simulink model "save_old_atan2"  (Simulink 7.6)
settings: Solver=ode45  StartTime=0.0  StopTime=10.0  RelTol=1e-3
libraries: simulink x14
settings Model: Creator=jporter  LastModifiedBy=jporter

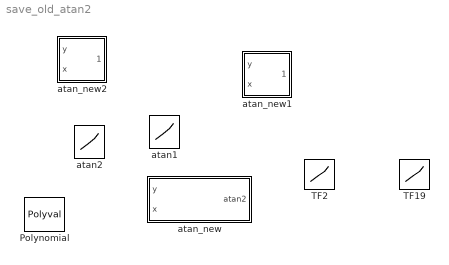
== system save_old_atan2 ==
  Polynomial : Polyval  Coefs=polyfit( [-100:100], atan( [-100:100] ), 12 )
  TF19 : Lookup  InputValues=[-5:5]  Table=atan([-5:5])  OutDataTypeStr=double
  TF2 : Lookup  InputValues=fi([-10 -5 -2.5:.1:-.11 -.1:.001:.1 .11:.1:2.5 5 10], 1, 32, 27)  Table=fi([ -pi/2 atan([-5 -2.5:.1:-.11 -.1:.001:.1 .11:.1:2.5 5]) pi/2 ], 1, 32, 30)  LookUpMeth=Interpolation-Use End Values  OutDataTypeStr=double
  atan1 : Lookup2D  RowIndex=[-0.0007 -7e-005 -7e-006 -7e-007 -7e-008 0 7e-008 7e-007 7e-006 7e-005 0.0007]  ColumnIndex=[-0.0004 -4e-005 -4e-006 -4e-007 -4e-008 0 4e-008 4e-007 4e-006 4e-005 0.0004]  Table=[-2.08994244104142 -1.62787710920116 -1.57651055031409 -1.57136775530413 -1.57085346965198 -1.5707963267949 -1.57073918393782 -1.57022489828566 -1.5650821032757 -1.51371554438863 -1.05165021254837;-2.96834698713743 -2.08994244104142 -1.62787710920116 -1.57651055031409 -1.57136775530413 -1.5707963267949 -1.57022489828566 -1.5650821032757 -1.51371554438863 -1.05165021254837 -0.173245666452365;-3.12409443971994 -2.96834698713743 -2.08994244104142 -1.62787710920116 -1.57651055031409 -1.5707963267949 -1.5650821032757 -1.51371554438863 -1.05165021254837 -0.173245666452365 -0.0174982138698566;-3.13984265537625 -3.12409443971994 -2.96834698713743 -2.08994244104142 -1.62787710920116 -1.5707963267949 -1.51371554438863 -1.05165021254837 -0.173245666452365 -0.0174982138698566 -0.00174999821354495;-3.14141765359158 -3.13984265537625 -3.12409443971994 -2.96834698713743 -2.08994244104142 -1.5707963267949 -1.05165021254837 -0.173245666452365 -0.0174982138698566 -0.00174999821354495 -0.000174999998213542;3.14159265358979 3.14159265358979 3.14159265358979 3.14159265358979 3.14159265358979 0 0 0 0 0 0;3.14141765359158 3.13984265537625 3.12409443971994 2.96834698713743 2.08994244104142 1.5707963267949 1.05165021254837 0.173245666452365 0.0174982138698566 0.00174999821354495 0.000174999998213542;3.13984265537625 3.12409443971994 2.96834698713743 2.08994244104142 1.62787710920116 1.5707963267949 1.51371554438863 1.05165021254837 0.173245666452365 0.0174982138698566 0.00174999821354495;3.12409443971994 2.96834698713743 2.08994244104142 1.62787710920116 1.57651055031409 1.5707963267949 1.5650821032757 1.51371554438863 1.05165021254837 0.173245666452365 0.0174982138698566;2.96834698713743 2.08994244104142 1.62787710920116 1.57651055031409 1.57136775530413 1.5707963267949 1.57022489828566 1.5650821032757 1.51371554438863 1.05165021254837 0.173245666452365;2.08994244104142 1.62787710920116 1.57651055031409 1.57136775530413 1.57085346965198 1.5707963267949 1.57073918393782 1.57022489828566 1.5650821032757 1.51371554438863 1.05165021254837]  OutDataTypeStr=fixdt(1,32,29)
  atan2 : Lookup2D  RowIndex=[0 1.26491106406735e-008 2e-008 4e-008 1.26491106406735e-007 2e-007 4e-007 1.26491106406735e-006 2e-006 4e-006 1.26491106406735e-005 2e-005 4e-005 0.000126491106406735 0.0002 0.0004]  ColumnIndex=[0.999999993 0.999999997786406 0.9999999993 0.999999999778641 0.99999999993 0.999999999977864 0.999999999993 0.999999999997786 0.9999999999993 0.999999999999779 1]  Table=[0 0 0 0 0 0 0 0 0 0 0;1.26491107292173e-008 1.26491106686735e-008 1.26491106495279e-008 1.26491106434735e-008 1.2649110641559e-008 1.26491106409535e-008 1.26491106407621e-008 1.26491106407015e-008 1.26491106406824e-008 1.26491106406763e-008 1.26491106406735e-008;2.000000014e-008 2.00000000442719e-008 2.0000000014e-008 2.00000000044272e-008 2.00000000014e-008 2.00000000004427e-008 2.000000000014e-008 2.00000000000443e-008 2.0000000000014e-008 2.00000000000044e-008 2e-008;4.000000028e-008 4.00000000885438e-008 4.0000000028e-008 4.00000000088544e-008 4.00000000028e-008 4.00000000008854e-008 4.000000000028e-008 4.00000000000885e-008 4.0000000000028e-008 4.00000000000088e-008 4e-008;1.26491107292172e-007 1.26491106686735e-007 1.26491106495278e-007 1.26491106434735e-007 1.26491106415589e-007 1.26491106409535e-007 1.2649110640762e-007 1.26491106407015e-007 1.26491106406823e-007 1.26491106406763e-007 1.26491106406735e-007;2.00000001399997e-007 2.00000000442716e-007 2.00000000139997e-007 2.00000000044269e-007 2.00000000013997e-007 2.00000000004425e-007 2.00000000001397e-007 2.0000000000044e-007 2.00000000000137e-007 2.00000000000042e-007 1.99999999999997e-007;4.00000002799979e-007 4.00000000885416e-007 4.00000000279979e-007 4.00000000088523e-007 4.00000000027979e-007 4.00000000008833e-007 4.00000000002779e-007 4.00000000000864e-007 4.00000000000259e-007 4.00000000000067e-007 3.99999999999979e-007;1.26491107292105e-006 1.26491106686668e-006 1.26491106495211e-006 1.26491106434668e-006 1.26491106415522e-006 1.26491106409468e-006 1.26491106407553e-006 1.26491106406948e-006 1.26491106406756e-006 1.26491106406696e-006 1.26491106406668e-006;2.00000001399733e-006 2.00000000442452e-006 2.00000000139733e-006 2.00000000044005e-006 2.00000000013733e-006 2.00000000004161e-006 2.00000000001133e-006 2.00000000000176e-006 1.99999999999873e-006 1.99999999999778e-006 1.99999999999733e-006;4.00000002797867e-006 4.00000000883304e-006 4.00000000277867e-006 4.00000000086411e-006 4.00000000025867e-006 4.00000000006721e-006 4.00000000000667e-006 3.99999999998752e-006 3.99999999998147e-006 3.99999999997955e-006 3.99999999997867e-006;1.26491107285427e-005 1.26491106679989e-005 1.26491106488533e-005 1.26491106427989e-005 1.26491106408843e-005 1.26491106402789e-005 1.26491106400874e-005 1.26491106400269e-005 1.26491106400078e-005 1.26491106400017e-005 1.26491106399989e-005;2.00000001373333e-005 2.00000000416052e-005 2.00000000113333e-005 2.00000000017605e-005 1.99999999987333e-005 1.99999999977761e-005 1.99999999974733e-005 1.99999999973776e-005 1.99999999973473e-005 1.99999999973378e-005 1.99999999973333e-005;4.00000002586667e-005 4.00000000672104e-005 4.00000000066667e-005 3.99999999875211e-005 3.99999999814667e-005 3.99999999795521e-005 3.99999999789467e-005 3.99999999787552e-005 3.99999999786947e-005 3.99999999786755e-005 3.99999999786667e-005;0.000126491106617554 0.000126491106012116 0.00012649110582066 0.000126491105760116 0.00012649110574097 0.000126491105734916 0.000126491105733001 0.000126491105732396 0.000126491105732205 0.000126491105732144 0.000126491105732116;0.000199999998733333 0.000199999997776052 0.000199999997473333 0.000199999997377605 0.000199999997347333 0.000199999997337761 0.000199999997334733 0.000199999997333776 0.000199999997333473 0.000199999997333378 0.000199999997333333;0.000399999981466668 0.000399999979552106 0.000399999978946669 0.000399999978755213 0.000399999978694669 0.000399999978675523 0.000399999978669469 0.000399999978667554 0.000399999978666949 0.000399999978666757 0.000399999978666669]  OutDataTypeStr=fixdt(1,32,42)
  atan_new : Subsystem
  atan_new1 : Subsystem
  atan_new2 : Subsystem

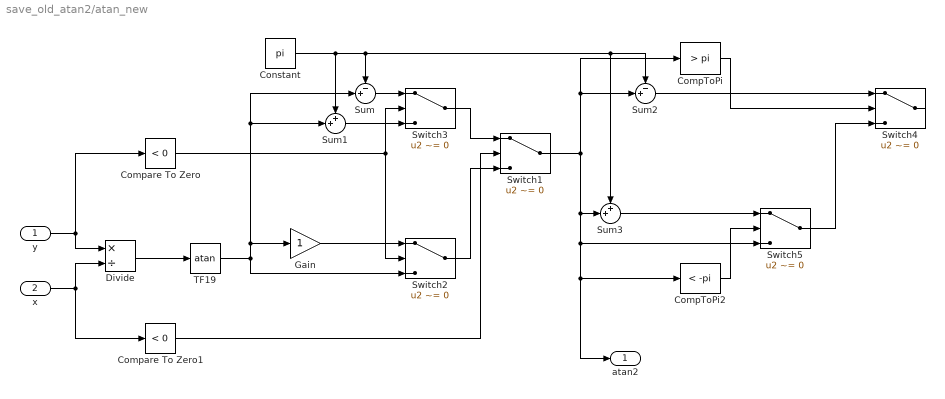
== system save_old_atan2/atan_new ==
  y : Inport
  x : Inport  Port=2
  CompToPi : simulink/Logic and Bit Operations/Compare To Constant  SystemSampleTime=-1  relop=>  const=pi  LogicOutDataTypeMode=uint8
  CompToPi2 : simulink/Logic and Bit Operations/Compare To Constant  SystemSampleTime=-1  relop=<  const=-pi  LogicOutDataTypeMode=uint8
  Compare To Zero : simulink/Logic and Bit Operations/Compare To Zero  SystemSampleTime=-1  relop=<  LogicOutDataTypeMode=uint8
  Compare To Zero1 : simulink/Logic and Bit Operations/Compare To Zero  SystemSampleTime=-1  relop=<  LogicOutDataTypeMode=uint8
  Constant : Constant  Value=pi
  Divide : Product  Inputs=*/
  Gain : Gain
  Sum : Sum  Inputs=-+|
  Sum1 : Sum  Inputs=++|
  Sum2 : Sum  Inputs=-+|
  Sum3 : Sum  Inputs=++|
  Switch{1..5} (5 alike) : Switch  Criteria=u2 ~= 0
  TF19 : Trigonometry  Operator=atan
  atan2 : Outport
  wires:
  Compare To Zero1/1 -> Switch1/2
  Compare To Zero/1 -> Switch2/2, Switch3/2
  Switch5/1 -> Switch4/3
  Sum3/1 -> Switch5/1
  Switch1/1 -> CompToPi/1, Sum2/2, atan2/1, CompToPi2/1, Switch5/3, Sum3/2
  Sum2/1 -> Switch4/1
  CompToPi2/1 -> Switch5/2
  CompToPi/1 -> Switch4/2
  Sum1/1 -> Switch3/3
  Sum/1 -> Switch3/1
  Constant/1 -> Sum3/1, Sum2/1, Sum/1, Sum1/1
  Gain/1 -> Switch2/1
  TF19/1 -> Sum1/2, Sum/2, Gain/1, Switch2/3
  Switch3/1 -> Switch1/1
  Switch2/1 -> Switch1/3
  Divide/1 -> TF19/1
  x/1 -> Compare To Zero1/1, Divide/2
  y/1 -> Compare To Zero/1, Divide/1

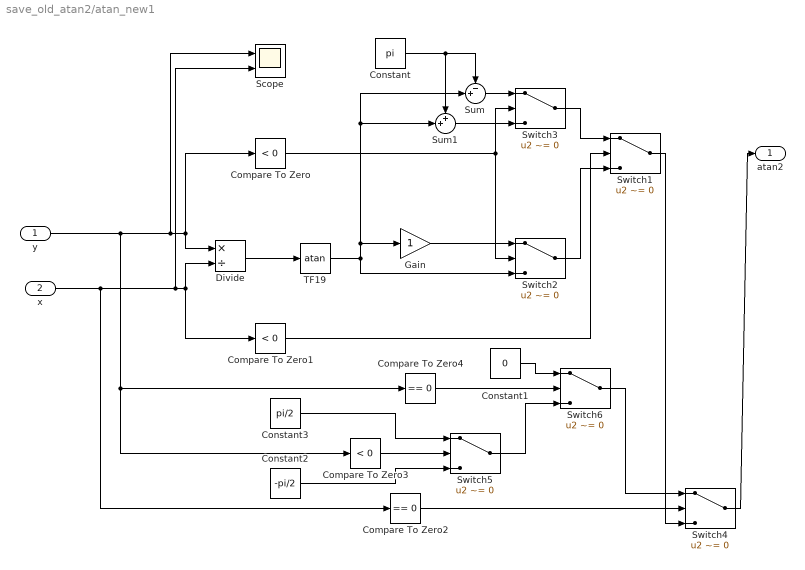
== system save_old_atan2/atan_new1 ==
  y : Inport
  x : Inport  Port=2
  Compare To Zero : simulink/Logic and Bit Operations/Compare To Zero  SystemSampleTime=-1  relop=<  LogicOutDataTypeMode=uint8
  Compare To Zero1 : simulink/Logic and Bit Operations/Compare To Zero  SystemSampleTime=-1  relop=<  LogicOutDataTypeMode=uint8
  Compare To Zero2 : simulink/Logic and Bit Operations/Compare To Zero  SystemSampleTime=-1  relop===  LogicOutDataTypeMode=uint8
  Compare To Zero3 : simulink/Logic and Bit Operations/Compare To Zero  SystemSampleTime=-1  relop=<  LogicOutDataTypeMode=uint8
  Compare To Zero4 : simulink/Logic and Bit Operations/Compare To Zero  SystemSampleTime=-1  relop===  LogicOutDataTypeMode=uint8
  Constant : Constant  Value=pi
  Constant1 : Constant  Value=0
  Constant2 : Constant  Value=-pi/2
  Constant3 : Constant  Value=pi/2
  Divide : Product  Inputs=*/
  Gain : Gain
  Scope : Scope  NumInputPorts=2
      settings: YMin=-5~-5  YMax=5~5  SaveName=ScopeData2
  Sum : Sum  Inputs=-+|
  Sum1 : Sum  Inputs=++|
  Switch{1..6} (6 alike) : Switch  Criteria=u2 ~= 0
  TF19 : Trigonometry  Operator=atan
  atan2 : Outport
  wires:
  y/1 -> Divide/1, Compare To Zero/1, Scope/1, Compare To Zero4/1, Compare To Zero3/1
  x/1 -> Divide/2, Compare To Zero1/1, Scope/2, Compare To Zero2/1
  Divide/1 -> TF19/1
  Switch2/1 -> Switch1/3
  Switch3/1 -> Switch1/1
  TF19/1 -> Switch2/3, Gain/1, Sum/2, Sum1/2
  Gain/1 -> Switch2/1
  Constant/1 -> Sum1/1, Sum/1
  Sum/1 -> Switch3/1
  Sum1/1 -> Switch3/3
  Compare To Zero/1 -> Switch3/2, Switch2/2
  Compare To Zero1/1 -> Switch1/2
  Compare To Zero2/1 -> Switch4/2
  Compare To Zero3/1 -> Switch5/2
  Compare To Zero4/1 -> Switch6/2
  Switch5/1 -> Switch6/3
  Constant1/1 -> Switch6/1
  Switch6/1 -> Switch4/1
  Switch1/1 -> Switch4/3
  Switch4/1 -> atan2/1
  Constant2/1 -> Switch5/3
  Constant3/1 -> Switch5/1

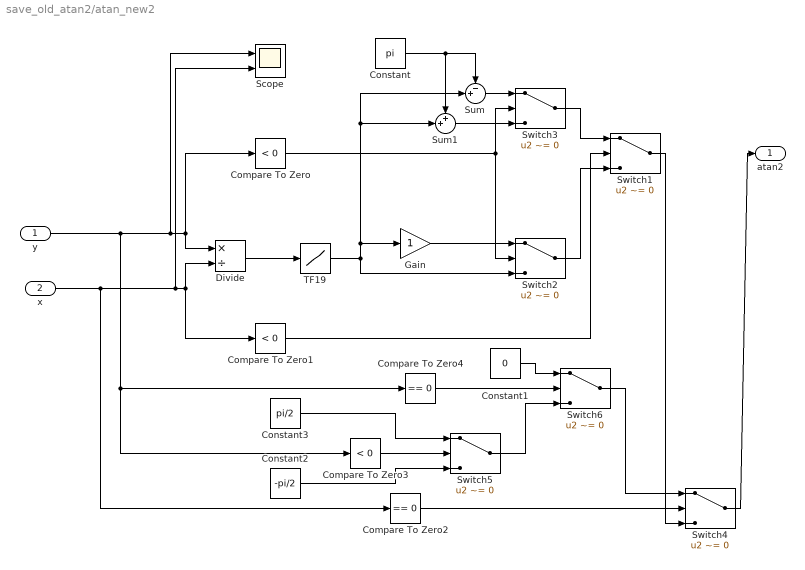
== system save_old_atan2/atan_new2 ==
  y : Inport
  x : Inport  Port=2
  Compare To Zero : simulink/Logic and Bit Operations/Compare To Zero  SystemSampleTime=-1  relop=<  LogicOutDataTypeMode=uint8
  Compare To Zero1 : simulink/Logic and Bit Operations/Compare To Zero  SystemSampleTime=-1  relop=<  LogicOutDataTypeMode=uint8
  Compare To Zero2 : simulink/Logic and Bit Operations/Compare To Zero  SystemSampleTime=-1  relop===  LogicOutDataTypeMode=uint8
  Compare To Zero3 : simulink/Logic and Bit Operations/Compare To Zero  SystemSampleTime=-1  relop=<  LogicOutDataTypeMode=uint8
  Compare To Zero4 : simulink/Logic and Bit Operations/Compare To Zero  SystemSampleTime=-1  relop===  LogicOutDataTypeMode=uint8
  Constant : Constant  Value=pi
  Constant1 : Constant  Value=0
  Constant2 : Constant  Value=-pi/2
  Constant3 : Constant  Value=pi/2
  Divide : Product  Inputs=*/
  Gain : Gain
  Scope : Scope  NumInputPorts=2
      settings: YMin=-5~-5  YMax=5~5  SaveName=ScopeData2
  Sum : Sum  Inputs=-+|
  Sum1 : Sum  Inputs=++|
  Switch{1..6} (6 alike) : Switch  Criteria=u2 ~= 0
  TF19 : Lookup  InputValues=[-5:5]  Table=atan([-5:5])
  atan2 : Outport
  wires:
  y/1 -> Divide/1, Compare To Zero/1, Scope/1, Compare To Zero4/1, Compare To Zero3/1
  x/1 -> Divide/2, Compare To Zero1/1, Scope/2, Compare To Zero2/1
  Divide/1 -> TF19/1
  Switch2/1 -> Switch1/3
  Switch3/1 -> Switch1/1
  TF19/1 -> Switch2/3, Gain/1, Sum/2, Sum1/2
  Gain/1 -> Switch2/1
  Constant/1 -> Sum1/1, Sum/1
  Sum/1 -> Switch3/1
  Sum1/1 -> Switch3/3
  Compare To Zero/1 -> Switch3/2, Switch2/2
  Compare To Zero1/1 -> Switch1/2
  Compare To Zero2/1 -> Switch4/2
  Compare To Zero3/1 -> Switch5/2
  Compare To Zero4/1 -> Switch6/2
  Switch5/1 -> Switch6/3
  Constant1/1 -> Switch6/1
  Switch6/1 -> Switch4/1
  Switch1/1 -> Switch4/3
  Switch4/1 -> atan2/1
  Constant2/1 -> Switch5/3
  Constant3/1 -> Switch5/1
